simulink model "Boost"  (R2014a)
settings: Solver=ode23tb  StartTime=0.0  StopTime=8e-3  RelTol=1e-3  AbsTol=1e-3
libraries: powerlib x8, powerlib_meascontrol x1
settings Model: CovSFcnEnable=on  ExtModeTrigMode=oneshot  ExtModeArmWhenConnect=off  ExtModeAutoUpdateStatusClock=off  Creator=dkennedy  LastModifiedBy=DELL
settings DataIOCC: LimitDataPoints=off  SignalLoggingSaveFormat=ModelDataLogs  SignalLoggingName=sigsOut
settings OptimizationCC: BlockReduction=off  BooleanDataType=off  InitFltsAndDblsToZero=on
settings DebuggingCC: SaveWithParameterizedLinksMsg=none  UnderspecifiedInitializationDetection=Classic  SignalResolutionControl=TryResolveAllWithWarning  SolverPrmCheckMsg=none  MultiTaskDSMMsg=warning  MultiTaskCondExecSysMsg=none  FcnCallInpInsideContextMsg=EnableAllAsWarning  FrameProcessingCompatibilityMsg=error
settings HardwareCC: TargetUnknown=on
settings GRTTargetCC: TargetFcnLib=ansi_tfl_tmw.mat  CombineOutputUpdateFcns=off  GRTInterface=on
settings ConfigurationSet: Description=Simscape Multibody

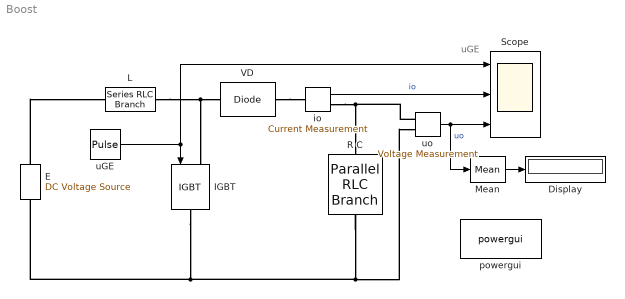
== system Boost ==
  note: uGE
  Display : Display
  E : powerlib/Electrical Sources/DC Voltage Source  Description=source block  Amplitude=100  Measurements=None
      settings: AttributesFormatString=%<Amplitude>V
  IGBT : powerlib/Power Electronics/IGBT  Ron=0.01  Lon=1e-6  Vf=1  Tf=1e-6  Tt=1e-6  IC=0  Rs=10000  Cs=inf  Measurements=off
      settings: AttributesFormatString=\n
  L : powerlib/Elements/Series RLC Branch  LConnTagsString=__new0  RConnTagsString=__new0  BranchType=L  Resistance=0  Inductance=1e-3  SetiL0=off  InitialCurrent=0  Capacitance=inf  Setx0=off  InitialVoltage=0  Measurements=None
  Mean : powerlib_meascontrol/Measurements/Mean  Freq=10000  Vinit=0  Ts=0  treatSBRowAsCol=off
  R C : powerlib/Elements/Parallel RLC Branch  LConnTagsString=a  RConnTagsString=__new0  BranchType=RC  Resistance=50  Inductance=inf  SetiL0=off  InitialCurrent=0  Capacitance=2e-5  Setx0=off  InitialVoltage=333.3  Measurements=None
  Scope : Scope  NumInputPorts=3
      settings: TimeRange=auto  MaxDataPoints=50000  SaveToWorkspace=off  SaveName=var  YMin=-0.125~-3.97878~-41.05527  YMax=1.125~35.80901~369.49746  SampleTime=-1
  VD : powerlib/Power Electronics/Diode  Ron=0.05  Lon=0.1e-6  Vf=0.8  IC=10  UseSnubber=0  Rs=inf  Cs=inf  Measurements=off
  io : powerlib/Measurements/Current Measurement  PhasorSimulation=off  OutputType=Complex  PSBequivalent=0
  powergui : powerlib/powergui  Priority=1  SimulationMode=Continuous  SampleTime=50e-6  frequency=60  Iterations=50  frequencyindice=0  Pbase=100e6  ErrMax=1e-4  UnitsV=kV  UnitsW=MW  buscounter=0  FunctionMessages=off  echomessages=off  EnableUseOfTLC=off  CurrentSourceSwitches=off  DisableSnubberDevices=off  DisableRonSwitches=off  DisableVfSwitches=off  DisplayEquations=off  AutomaticDiscreteSolvers=off  SolverType=Tustin/Backward Euler (TBE)  Interpol=off  ExternalGateDelay=off  methode=off  Ts=100  x0status=blocks  SPID=on  SwTol=0  HookPort=off  NonlinearTolerance=1e-4  nMaxIteration=100  ContinueOnMaxIteration=off  RestoreLinks=warning  ResistiveCurrentMeasurement=off  Frange=[0:2:500]  Ylog=off  Xlog=on  ShowGrid=off  save=off  variable=ZData  structure=0  ZoomFFT=off  StartTime=0.0  cycles=1  DisplayStyle=1  fundamental=60  FreqAxis=off  MaxFrequency=1000  frequencyindicesteady=1  RmsSteady=1  display=off
  uGE : DiscretePulseGenerator  PulseType=Time based  Period=1e-4  PulseWidth=50
  uo : powerlib/Measurements/Voltage Measurement  Tag=PoWeRsYsTeMmEaSuReMeNt  PhasorSimulation=off  OutputType=Magnitude  PSBequivalent=0
  wires:
  io/1 -> Scope/2  "io"
  uGE/1 -> IGBT/1, Scope/1
  Mean/1 -> Display/1
  uo/1 -> Mean/1, Scope/3  "uo"
  connections:
  uo/LConn1 -- R C/LConn1 -- io/RConn1
  R C/RConn1 -- uo/LConn2 -- IGBT/RConn1 -- E/LConn1
  E/RConn1 -- L/LConn1
  L/RConn1 -- VD/LConn1 -- IGBT/LConn1
  VD/RConn1 -- io/LConn1
